simulink model "DCSVA_Project"  (R2019a)
settings: Solver=ode45  StartTime=0.0  StopTime=10  RelTol=1e-3  EnableMultiTasking=on
libraries: fuzblock x1
settings Model: Creator=VICTOR  LastModifiedBy=krish
settings SolverCC: ZeroCrossAlgorithm=Non-adaptive
settings DataIOCC: LimitDataPoints=on  SaveFormat=Array  SignalLoggingSaveFormat=ModelDataLogs  ReturnWorkspaceOutputs=off
settings OptimizationCC: ExpressionDepthLimit=2147483647  InitFltsAndDblsToZero=on  LifeSpan=inf
settings DebuggingCC: UnderspecifiedInitializationDetection=Classic  MergeDetectMultiDrivingBlocksExec=none  SolverPrmCheckMsg=warning  FcnCallInpInsideContextMsg=warning  StateNameClashWarn=warning  SFUnexpectedBacktrackingDiag=warning  SFNoUnconditionalDefaultTransitionDiag=warning  SFExecutionAtInitializationDiag=none  ArithmeticOperatorsInVariantConditions=warning
settings HardwareCC: ProdBitPerPointer=32  ProdBitPerSizeT=32  ProdBitPerPtrDiffT=32  ProdLargestAtomicFloat=None  ProdIntDivRoundTo=Undefined  ProdEndianess=Unspecified  ProdWordSize=32  ProdHWDeviceType=32-bit Generic
settings ModelReferenceCC: PropagateSignalLabelsOutOfModel=off
settings CodeAppCC: StateflowObjectComments=on
settings GRTTargetCC: TargetLangStandard=C89/C90 (ANSI)  CombineOutputUpdateFcns=off  GRTInterface=on
settings ConfigComp: CovMetricSettings=dw  CovHtmlReporting=on  CovSaveCumulativeToWorkspaceVar=on  CovSaveSingleToWorkspaceVar=on

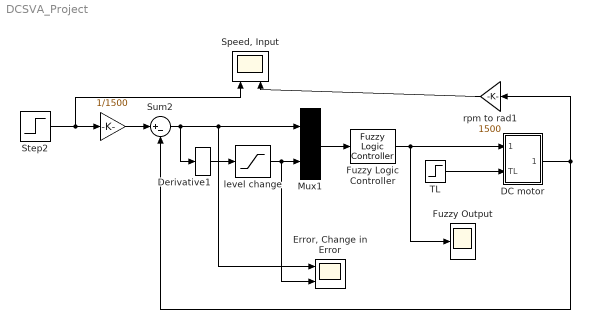
== system DCSVA_Project ==
  " " : Gain  Gain=1/1500
  DC motor : Subsystem  mask{Ra=1, La=0.5, J=0.01, D=0.1}
      mask prompts: Ra "Armature Resistance (Ra)"; La "Armature Inductance (La)"; J "Inertia (J)"; D "Damping (B)"
  Derivative1 : Derivative
  "Error, Change in Error" : Scope  NumInputPorts=2
  "Fuzzy Logic Controller " : fuzblock/Fuzzy Logic  Controller  FIS='control.fis'  OutputSampleNumber=101  DataType=double  FuzzifiedInputs=off  RuleFiringStrengths=off  RuleOutputs=off  AggregatedOutputs=off  SimulateUsing=Interpreted execution  OutOfRangeInputValueMessage=warning  NoRuleFiredMessage=warning  EmptyOutputFuzzySetMessage=warning
  Fuzzy Output : Scope
  Mux1 : Mux  Inputs=2
  "Speed, Input" : Scope  NumInputPorts=2
  Step2 : Step  Time=5  Before=800  After=1450  SampleTime=0.001
  Sum2 : Sum  Inputs=|+-
  TL : Step  Time=7  Before=0.0001  After=0.002  SampleTime=0
  level change : Saturate  UpperLimit=2  LowerLimit=-2
  rpm to rad1 : Gain  Gain=1500
  wires:
  Sum2/1 -> Derivative1/1, "Error, Change in Error"/1, Mux1/1
  Mux1/1 -> "Fuzzy Logic Controller "/1
  Step2/1 -> "Speed, Input"/1, " "/1
  rpm to rad1/1 -> "Speed, Input"/2
  " "/1 -> Sum2/1
  TL/1 -> DC motor/2(TL)
  Derivative1/1 -> level change/1
  DC motor/1(Out1) -> rpm to rad1/1, Sum2/2
  "Fuzzy Logic Controller "/1 -> DC motor/1(In1), Fuzzy Output/1
  level change/1 -> "Error, Change in Error"/2, Mux1/2

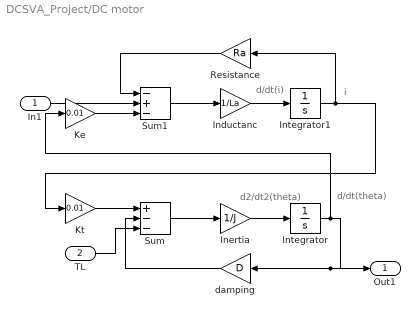
== system DCSVA_Project/DC motor ==
  note: d/dt(i)
  note: i
  note: d/dt(theta)
  note: d2/dt2(theta)
  In1 : Inport
  TL : Inport  Port=2
  Inductanc : Gain  Gain=1/La  SaturateOnIntegerOverflow=on  OutDataTypeStr=Inherit: Same as input  ParamDataTypeStr=Inherit: Same as input
  Inertia : Gain  Gain=1/J  SaturateOnIntegerOverflow=on  OutDataTypeStr=Inherit: Same as input  ParamDataTypeStr=Inherit: Same as input
  Integrator : Integrator
  Integrator1 : Integrator
  Ke : Gain  Gain=0.01  SaturateOnIntegerOverflow=on  OutDataTypeStr=Inherit: Same as input  ParamDataTypeStr=Inherit: Same as input
  Kt : Gain  Gain=0.01  SaturateOnIntegerOverflow=on  OutDataTypeStr=Inherit: Same as input  ParamDataTypeStr=Inherit: Same as input
  Resistance : Gain  Gain=Ra  SaturateOnIntegerOverflow=on  OutDataTypeStr=Inherit: Same as input  ParamDataTypeStr=Inherit: Same as input
  Sum : Sum  Inputs=+--  SaturateOnIntegerOverflow=on  InputSameDT=on  OutDataTypeStr=Inherit: Same as first input
  Sum1 : Sum  Inputs=-+-  SaturateOnIntegerOverflow=on  InputSameDT=on  OutDataTypeStr=Inherit: Same as first input
  damping : Gain  Gain=D  SaturateOnIntegerOverflow=on  OutDataTypeStr=Inherit: Same as input  ParamDataTypeStr=Inherit: Same as input
  Out1 : Outport
  wires:
  Integrator1/1 -> Resistance/1, Kt/1
  Integrator/1 -> Ke/1, damping/1, Out1/1
  Ke/1 -> Sum1/3
  Resistance/1 -> Sum1/1
  Kt/1 -> Sum/1
  damping/1 -> Sum/2
  Sum1/1 -> Inductanc/1
  Sum/1 -> Inertia/1
  Inertia/1 -> Integrator/1
  Inductanc/1 -> Integrator1/1
  In1/1 -> Sum1/2
  TL/1 -> Sum/3
